simulink model "cyclo"  (R2020a)
settings: Solver=VariableStepAuto  StartTime=0.0  StopTime=inf  RelTol=1e-3
model workspace (MAT data in the model file):
  f = 50
  m = 3
libraries: powerlib x13
settings Model: Creator=snehk  LastModifiedBy=snehk

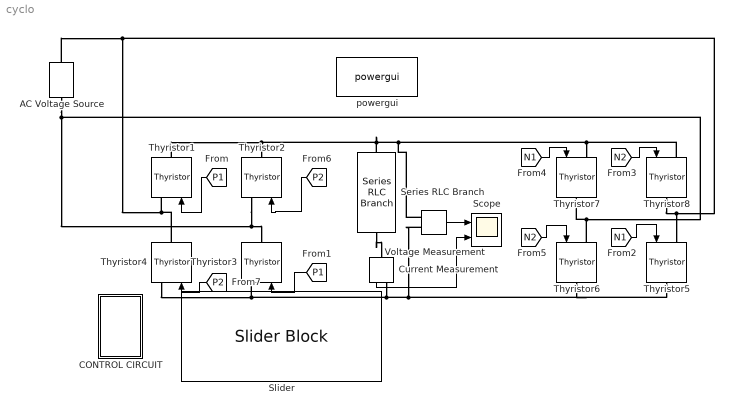
== system cyclo ==
  AC Voltage Source : powerlib/Electrical Sources/AC Voltage Source  Amplitude=230  Phase=0  Frequency=50  SampleTime=0  Measurements=None  BusType=swing  Pref=10e3  Qref=0  Qmin=-inf  Qmax=+inf
  CONTROL CIRCUIT : Subsystem
  Current Measurement : powerlib/Measurements/Current Measurement  PhasorSimulation=off  OutputType=Complex  PSBequivalent=0
  Scope : Scope  NumInputPorts=2
  Series RLC Branch : powerlib/Elements/Series RLC Branch  LConnTagsString=__new0  RConnTagsString=__new0  BranchType=RL  Resistance=100  Inductance=0.1  SetiL0=off  InitialCurrent=0  Capacitance=1e-6  Setx0=off  InitialVoltage=0  Measurements=None
  Slider : SliderBlock  LabelPosition=Bottom  ScaleMax=180
  Thyristor{1..8} (8 alike) : powerlib/Power Electronics/Thyristor  Ron=0.1  Lon=0  Vf=0  IC=0  Rs=500  Cs=250e-9  Measurements=off
  Voltage Measurement : powerlib/Measurements/Voltage Measurement  PhasorSimulation=off  OutputType=Complex  PSBequivalent=0
  powergui : powerlib/powergui  Priority=1  SimulationMode=Continuous  SampleTime=1e-4  frequency=60  Iterations=50  frequencyindice=50  Pbase=100e6  ErrMax=1e-4  UnitsV=kV  UnitsW=MW  buscounter=0  FunctionMessages=off  echomessages=off  EnableUseOfTLC=off  CurrentSourceSwitches=off  DisableSnubberDevices=off  DisableRonSwitches=off  DisableVfSwitches=off  DisplayEquations=off  AutomaticDiscreteSolvers=off  SolverType=Tustin/Backward Euler (TBE)  Interpol=off  ExternalGateDelay=off  methode=off  Ts=100  x0status=blocks  SPID=on  SwTol=0  HookPort=off  NonlinearTolerance=1e-4  nMaxIteration=100  ContinueOnMaxIteration=off  RestoreLinks=warning  ResistiveCurrentMeasurement=off  Frange=[0:2:500]  Ylog=off  Xlog=on  ShowGrid=off  save=off  variable=ZData  structure=0  ZoomFFT=off  StartTime=0.0  cycles=1  DisplayStyle=1  fundamental=60  FreqAxis=off  MaxFrequency=1000  frequencyindicesteady=1  RmsSteady=1  display=off
  wires:
  [P1] -> Thyristor1/1
  [P1] -> Thyristor3/1
  [P2] -> Thyristor4/1
  [P2] -> Thyristor2/1
  [N2] -> Thyristor8/1
  [N1] -> Thyristor7/1
  Voltage Measurement/1 -> Scope/1
  Current Measurement/1 -> Scope/2
  [N2] -> Thyristor6/1
  [N1] -> Thyristor5/1
  connections:
  Thyristor8/RConn1 -- AC Voltage Source/RConn1 -- Thyristor1/LConn1 -- Thyristor4/RConn1 -- Thyristor5/LConn1
  Thyristor6/LConn1 -- Thyristor2/LConn1 -- Thyristor3/RConn1 -- AC Voltage Source/LConn1 -- Thyristor7/RConn1
  Thyristor4/LConn1 -- Current Measurement/RConn1 -- Thyristor6/RConn1 -- Thyristor5/RConn1 -- Voltage Measurement/LConn2 -- Thyristor3/LConn1
  Thyristor8/LConn1 -- Voltage Measurement/LConn1 -- Series RLC Branch/LConn1 -- Thyristor2/RConn1 -- Thyristor1/RConn1 -- Thyristor7/LConn1
  Series RLC Branch/RConn1 -- Current Measurement/LConn1

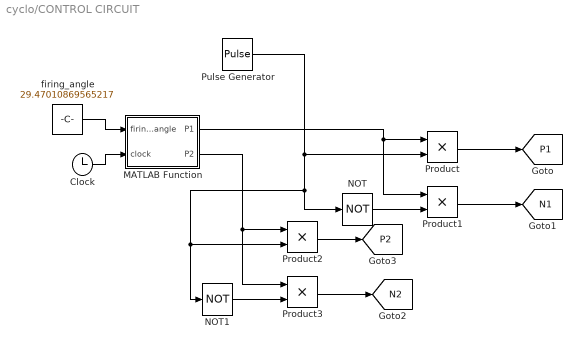
== system cyclo/CONTROL CIRCUIT ==
  Clock : Clock
  MATLAB Function : MATLAB Function  TreatAsAtomicUnit=on
  NOT : Logic  Operator=NOT  IconShape=distinctive  AllPortsSameDT=off  OutDataTypeStr=boolean
  NOT1 : Logic  Operator=NOT  IconShape=distinctive  AllPortsSameDT=off  OutDataTypeStr=boolean
  Product{,1..3} (4 alike) : Product
  Pulse Generator : DiscretePulseGenerator  PulseType=Time based  Period=2*m/f  PulseWidth=50
  firing_angle : Constant  Value=29.47010869565217
  tag scope: N1=global, N2=global, P1=global, P2=global
  wires:
  MATLAB Function/1(P1) -> Product1/1, Product/1
  Clock/1 -> MATLAB Function/2(clock)
  NOT/1 -> Product1/2
  firing_angle/1 -> MATLAB Function/1(firing_angle)
  NOT1/1 -> Product3/2
  Pulse Generator/1 -> NOT1/1, Product2/2, NOT/1, Product/2
  MATLAB Function/2(P2) -> Product3/1, Product2/1
  Product/1 -> [P1]
  Product3/1 -> [N2]
  Product2/1 -> [P2]
  Product1/1 -> [N1]

== matlab function cyclo/CONTROL CIRCUIT/MATLAB Function ==
  data: firing_angle input; P1 output; P2 output; clock input
function [P1, P2] = fcn(firing_angle, clock)
f = 50;
m = 3;
tt1 = 1/(2*f);
t = mod(clock,(1/(f)));
a = firing_angle/180;

if (t < (tt1))
    if (t > (a*tt1))
        a1 = 1;
        a2 = 0;
    else
        a1 = 0;
        a2 = 0;
    end
else
    if (t > (a*tt1 + 1/(2*f)))
        a2 = 1;
        a1 = 0;
    else
        a1 = 0;
        a2 = 0;
    end
end

P1 = a1;
P2 = a2;
